simulink model "m22"  (R2013b)
settings: Solver=ode45  StartTime=0.0  StopTime=30000  MaxStep=0.5  RelTol=1e-3
libraries: simulink x2
settings Model: Creator=user  LastModifiedBy=user

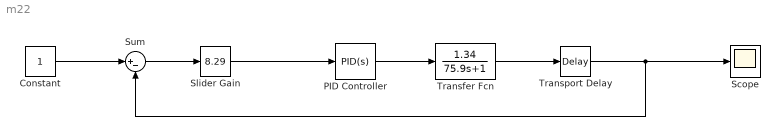
== system m22 ==
  Constant : Constant
  PID Controller : simulink/Continuous/PID Controller  Controller=PID  TimeDomain=Continuous-time  SampleTime=1  IntegratorMethod=Forward Euler  FilterMethod=Forward Euler  Form=Parallel  P=1  I=0  D=0  N=100  InitialConditionSource=internal  InitialConditionForIntegrator=0  InitialConditionForFilter=0  ExternalReset=none  LimitOutput=on  UpperSaturationLimit=16  LowerSaturationLimit=0  LinearizeAsGain=on  AntiWindupMode=none  Kb=1  TrackingMode=off  Kt=1  PParamMin=[]  PParamMax=[]  IParamMin=[]  IParamMax=[]  DParamMin=[]  DParamMax=[]  NParamMin=[]  NParamMax=[]  KbParamMin=[]  KbParamMax=[]  KtParamMin=[]  KtParamMax=[]  POutMin=[]  POutMax=[]  IOutMin=[]  IOutMax=[]  DOutMin=[]  DOutMax=[]  NOutMin=[]  NOutMax=[]  KbOutMin=[]  KbOutMax=[]  KtOutMin=[]  KtOutMax=[]  IntegratorOutMin=[]  IntegratorOutMax=[]  FilterOutMin=[]  FilterOutMax=[]  SumOutMin=[]  SumOutMax=[]  SumI1OutMin=[]  SumI1OutMax=[]  SumI2OutMin=[]  SumI2OutMax=[]  SumI3OutMin=[]  SumI3OutMax=[]  SumDOutMin=[]  SumDOutMax=[]  SaturationOutMin=[]  SaturationOutMax=[]  IntegratorContinuousStateAttributes=''  IntegratorStateMustResolveToSignalObject=off  IntegratorRTWStateStorageClass=Auto  FilterContinuousStateAttributes=''  FilterStateMustResolveToSignalObject=off  FilterRTWStateStorageClass=Auto
  Scope : Scope
      settings: TimeRange=106.6827697262479  YMin=0.9063380281690141  YMax=0.9265727699530517
  Slider Gain : simulink/Math Operations/Slider Gain  low=0  gain=8.29  high=10
  Sum : Sum  Inputs=|+-
  Transfer Fcn : TransferFcn  Numerator=[1.34]  Denominator=[75.9,1]
  Transport Delay : TransportDelay  DelayTime=11.4
  wires:
  Constant/1 -> Sum/1
  Sum/1 -> Slider Gain/1
  Slider Gain/1 -> PID Controller/1
  PID Controller/1 -> Transfer Fcn/1
  Transfer Fcn/1 -> Transport Delay/1
  Transport Delay/1 -> Sum/2, Scope/1
